simulink model "FOC_control"  (R2019a)
settings: Solver=VariableStepAuto  StartTime=0.0  StopTime=10.0  RelTol=1e-3
undefined symbols (not defined in the file or in its folder): PWM_EN, sf, Ts
libraries: nesl_utility x13, ee_lib x10, fl_lib x10, msbAdcArchitectures x6, eeTransforms x4, eePmsmCurrentController x1, eePmsmCurrentReferenceGen x1, eePwmGeneratorTwoLevel x1, eeVelocityController x1, simulink x1
(part 1 of 3)
settings Model: Creator=matthew  LastModifiedBy=matthew
settings DataIOCC: ReturnWorkspaceOutputs=off
settings DebuggingCC: ArithmeticOperatorsInVariantConditions=warning

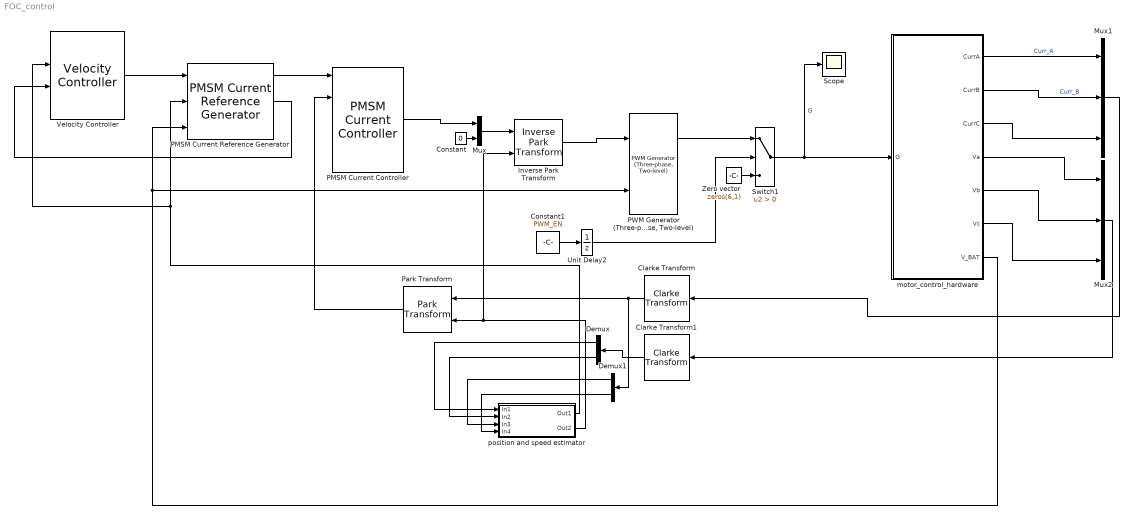
== system FOC_control ==
  Clarke Transform : eeTransforms/Clarke Transform  PowerInvariant=off
      settings: SourceProductName=Simscape Electrical  SourceProductBaseCode=PS
  Clarke Transform1 : eeTransforms/Clarke Transform  PowerInvariant=off
      settings: SourceProductName=Simscape Electrical  SourceProductBaseCode=PS
  Constant : Constant  Value=0  SampleTime=.00001
  Constant1 : Constant  Value=PWM_EN
  Demux : Demux  Outputs=2
  Demux1 : Demux  Outputs=2
  Inverse Park Transform : eeTransforms/Inverse Park Transform  AxisAlignment=Q-axis  PowerInvariant=off
      settings: SourceProductName=Simscape Electrical
  Mux : Mux  Inputs=2
  Mux1 : Mux  Inputs=3
  Mux2 : Mux  Inputs=3
  PMSM Current Controller : eePmsmCurrentController/PMSM Current Controller  Kp_id=1  Ki_id=100  Kaw_id=1  Kp_iq=1  Ki_iq=100  Kaw_iq=1  Ts=-1  Tsd=0.001  AxisPrio=Q-axis  ActZC=off  ActFF=on
      settings: SourceProductName=Simscape Electrical  SourceProductBaseCode=PS
  PMSM Current Reference Generator : eePmsmCurrentReferenceGen/PMSM Current Reference Generator  Vnom=300  Pmax=30000  Tmax=250  Ts=-1  RefType=Zero d-axis control  rpmVec=[0, 3000]  TqVec=[-100, 0, 100]  VdcVec=[300, 350]  idMatrix=zeros(2,3,2)  iqMatrix=zeros(2,3,2)  p=8  psim=0.04  Ld=0.00024  Lq=0.00029  Rs=0.01  RefExpEnable=0
      settings: SourceProductName=Simscape Electrical  SourceProductBaseCode=PS
  "PWM Generator (Three-phase, Two-level)" : eePwmGeneratorTwoLevel/PWM Generator (Three-phase, Two-level)  PWMMode=Continuous PWM (CPWM)  CPWMMode=SVM: space vector modulation  DPWMMode=60 DPWM: 60 degree discontinuous PWM  fsw=10000  Ts=Ts
      settings: SourceProductName=Simscape Electrical  SourceProductBaseCode=PS
  Park Transform : eeTransforms/Park Transform  AxisAlignment=Q-axis  PowerInvariant=off
      settings: SourceProductName=Simscape Electrical
  Scope : Scope
  Switch1 : Switch  Criteria=u2 > Threshold
  Unit Delay2 : UnitDelay  SampleTime=Ts  HasFrameUpgradeWarning=on
  Velocity Controller : eeVelocityController/Velocity Controller  CtrlType=PI control  Kp_w=1  Ki_w=1  Kv_w=1  Kaw_w=1  Ts=-1  Tsd=0.001  ActZC=off
      settings: SourceProductName=Simscape Electrical  SourceProductBaseCode=PS
  Zero vector : Constant  Value=zeros(6,1)  SampleTime=sf
  "motor_control_hardware " : Subsystem
  "position and speed estimator " : Subsystem
  wires:
  PMSM Current Reference Generator/1 -> PMSM Current Controller/1
  PMSM Current Controller/1 -> Mux/1
  Inverse Park Transform/1 -> "PWM Generator (Three-phase, Two-level)"/1
  Mux/1 -> Inverse Park Transform/1
  "PWM Generator (Three-phase, Two-level)"/1 -> Switch1/1
  Unit Delay2/1 -> Switch1/2
  Constant/1 -> Mux/2
  Zero vector/1 -> Switch1/3
  Switch1/1 -> Scope/1, "motor_control_hardware "/1(G)  "G"
  Velocity Controller/1 -> PMSM Current Reference Generator/1
  Mux1/1 -> Clarke Transform/1
  "motor_control_hardware "/1("CurrA ") -> Mux1/1  "Curr_A"
  "motor_control_hardware "/2("CurrB ") -> Mux1/2  "Curr_B"
  Park Transform/1 -> PMSM Current Controller/2
  Clarke Transform/1 -> Demux1/1, Park Transform/1
  "motor_control_hardware "/3("CurrC ") -> Mux1/3
  "motor_control_hardware "/4("Va ") -> Mux2/1
  "motor_control_hardware "/5("Vb ") -> Mux2/2
  "motor_control_hardware "/6("Vc ") -> Mux2/3
  Mux2/1 -> Clarke Transform1/1
  Clarke Transform1/1 -> Demux/1
  "position and speed estimator "/1(Out1) -> Velocity Controller/2, PMSM Current Reference Generator/2
  "position and speed estimator "/2(Out2) -> Inverse Park Transform/2, Park Transform/2
  "motor_control_hardware "/7("V_BAT ") -> "PWM Generator (Three-phase, Two-level)"/2, PMSM Current Reference Generator/3
  PMSM Current Reference Generator/2 -> Velocity Controller/3
  Demux/1 -> "position and speed estimator "/1(In1)
  Demux/2 -> "position and speed estimator "/2(In2)
  Demux1/1 -> "position and speed estimator "/3(In3)
  Demux1/2 -> "position and speed estimator "/4(In4)
  Constant1/1 -> Unit Delay2/1
